simulink model "simulinkm2"  (R2020b)
settings: Solver=VariableStepAuto  StartTime=0.0  StopTime=10.0  RelTol=1e-3
(part 3 of 5)

== matlab function simulinkm2/MATLAB Function2 ==
  data: q input; V_F output; q_dot input
 function V_F = forward_velocity_kinematics(q, q_dot)
    
    q1 = q(1)
     q2 = q(2)
     q3 = q(3)
     q4 = q(4)
     q5 = q(5)
     q6 = q(6)
    JM = [ 10*sin((pi*q5)/180)*(cos((pi*q1)/180)*sin((pi*q4)/180) - cos((pi*q2)/180)*cos((pi*q3)/180)*cos((pi*q4)/180)*sin((pi*q1)/180) + cos((pi*q4)/180)*sin((pi*q1)/180)*sin((pi*q2)/180)*sin((pi*q3)/180)) - 5*cos((pi*q2)/180)*sin((pi*q1)/180) - 5*sin((pi*q1)/180) - 10*cos((pi*q2)/180)*sin((pi*q1)/180)*sin((pi*q3)/180) - 10*cos((pi*q3)/180)*sin((pi*q1)/180)*sin((pi*q2)/180) - 10*sin((pi*(q2 + q3))/180)*cos((pi*q5)/180)*sin((pi*q1)/180),                                                                                                                                                                                                                                                                                                                                                                                                                                                                                                                                                                                                                                                                  cos((pi*q1)/180)*(10*cos((pi*(q2 + q3))/180) - 5*sin((pi*q2)/180) - 5*sin((pi*(q2 + q3))/180)*sin((pi*(q4 + q5))/180) + 10*cos((pi*(q2 + q3))/180)*cos((pi*q5)/180) + 5*sin((pi*(q2 + q3))/180)*sin((pi*(q4 - q5))/180)),                                                                                                                                                                                                                                                                                                                                                                                                                                                                                                                                                                                                                                                                                                                                                                                                                         cos((pi*q1)/180)*(10*cos((pi*(q2 + q3))/180) - 5*sin((pi*(q2 + q3))/180)*sin((pi*(q4 + q5))/180) + 10*cos((pi*(q2 + q3))/180)*cos((pi*q5)/180) + 5*sin((pi*(q2 + q3))/180)*sin((pi*(q4 - q5))/180)),                                                                                                                                                                                                                                                                                                                           cos((pi*(q2 + q3))/180)*(5*sin((pi*q1)/180) + 5*cos((pi*q2)/180)*sin((pi*q1)/180) - 5*sin((pi*q1)/180)*(cos((pi*q2)/180) + 1) - 10*sin((pi*q5)/180)*(cos((pi*q1)/180)*sin((pi*q4)/180) - cos((pi*q2)/180)*cos((pi*q3)/180)*cos((pi*q4)/180)*sin((pi*q1)/180) + cos((pi*q4)/180)*sin((pi*q1)/180)*sin((pi*q2)/180)*sin((pi*q3)/180)) + 10*cos((pi*q2)/180)*sin((pi*q1)/180)*sin((pi*q3)/180) + 10*cos((pi*q3)/180)*sin((pi*q1)/180)*sin((pi*q2)/180) + 10*sin((pi*(q2 + q3))/180)*cos((pi*q5)/180)*sin((pi*q1)/180)) - sin((pi*(q2 + q3))/180)*sin((pi*q1)/180)*(10*cos((pi*(q2 + q3))/180) - 5*sin((pi*(q2 + q3))/180)*sin((pi*(q4 + q5))/180) + 10*cos((pi*(q2 + q3))/180)*cos((pi*q5)/180) + 5*sin((pi*(q2 + q3))/180)*sin((pi*(q4 - q5))/180)),                                                                                                                                                                                                                                                                                                                                                                                                                                                                                           (cos((pi*q1)/180)*cos((pi*q4)/180) - sin((pi*q4)/180)*(sin((pi*q1)/180)*sin((pi*q2)/180)*sin((pi*q3)/180) - cos((pi*q2)/180)*cos((pi*q3)/180)*sin((pi*q1)/180)))*(10*cos((pi*(q2 + q3))/180)*cos((pi*q5)/180) - 5*sin((pi*(q2 + q3))/180)*sin((pi*(q4 + q5))/180) + 5*sin((pi*(q2 + q3))/180)*sin((pi*(q4 - q5))/180)) + sin((pi*(q2 + q3))/180)*sin((pi*q4)/180)*(5*sin((pi*q1)/180) + 5*cos((pi*q2)/180)*sin((pi*q1)/180) - 5*sin((pi*q1)/180)*(2*sin((pi*(q2 + q3))/180) + cos((pi*q2)/180) + 1) - 10*sin((pi*q5)/180)*(cos((pi*q1)/180)*sin((pi*q4)/180) - cos((pi*q2)/180)*cos((pi*q3)/180)*cos((pi*q4)/180)*sin((pi*q1)/180) + cos((pi*q4)/180)*sin((pi*q1)/180)*sin((pi*q2)/180)*sin((pi*q3)/180)) + 10*cos((pi*q2)/180)*sin((pi*q1)/180)*sin((pi*q3)/180) + 10*cos((pi*q3)/180)*sin((pi*q1)/180)*sin((pi*q2)/180) + 10*sin((pi*(q2 + q3))/180)*cos((pi*q5)/180)*sin((pi*q1)/180)),                                                                                                                                                                                                                                                                                                                                                                                                                                                                                                                                                                             (cos((pi*(q2 + q3))/180)*cos((pi*q5)/180) - sin((pi*(q2 + q3))/180)*cos((pi*q4)/180)*sin((pi*q5)/180))*(5*sin((pi*q1)/180) + 5*cos((pi*q2)/180)*sin((pi*q1)/180) - 5*sin((pi*q1)/180)*(2*sin((pi*(q2 + q3))/180) + cos((pi*q2)/180) + 1) - 10*sin((pi*q5)/180)*(cos((pi*q1)/180)*sin((pi*q4)/180) - cos((pi*q2)/180)*cos((pi*q3)/180)*cos((pi*q4)/180)*sin((pi*q1)/180) + cos((pi*q4)/180)*sin((pi*q1)/180)*sin((pi*q2)/180)*sin((pi*q3)/180)) + 10*cos((pi*q2)/180)*sin((pi*q1)/180)*sin((pi*q3)/180) + 10*cos((pi*q3)/180)*sin((pi*q1)/180)*sin((pi*q2)/180) + 10*sin((pi*(q2 + q3))/180)*cos((pi*q5)/180)*sin((pi*q1)/180)) + (sin((pi*q5)/180)*(cos((pi*q4)/180)*(sin((pi*q1)/180)*sin((pi*q2)/180)*sin((pi*q3)/180) - cos((pi*q2)/180)*cos((pi*q3)/180)*sin((pi*q1)/180)) + cos((pi*q1)/180)*sin((pi*q4)/180)) - cos((pi*q5)/180)*(cos((pi*q2)/180)*sin((pi*q1)/180)*sin((pi*q3)/180) + cos((pi*q3)/180)*sin((pi*q1)/180)*sin((pi*q2)/180)))*(10*cos((pi*(q2 + q3))/180)*cos((pi*q5)/180) - 5*sin((pi*(q2 + q3))/180)*sin((pi*(q4 + q5))/180) + 5*sin((pi*(q2 + q3))/180)*sin((pi*(q4 - q5))/180));
 5*cos((pi*q1)/180) + 5*cos((pi*q1)/180)*cos((pi*q2)/180) + 10*sin((pi*q5)/180)*(sin((pi*q1)/180)*sin((pi*q4)/180) + cos((pi*q1)/180)*cos((pi*q2)/180)*cos((pi*q3)/180)*cos((pi*q4)/180) - cos((pi*q1)/180)*cos((pi*q4)/180)*sin((pi*q2)/180)*sin((pi*q3)/180)) + 10*sin((pi*(q2 + q3))/180)*cos((pi*q1)/180)*cos((pi*q5)/180) + 10*cos((pi*q1)/180)*cos((pi*q2)/180)*sin((pi*q3)/180) + 10*cos((pi*q1)/180)*cos((pi*q3)/180)*sin((pi*q2)/180),                                                                                                                                                                                                                                                                                                                                                                                                                                                                                                                                                                                                                                                                  sin((pi*q1)/180)*(10*cos((pi*(q2 + q3))/180) - 5*sin((pi*q2)/180) - 5*sin((pi*(q2 + q3))/180)*sin((pi*(q4 + q5))/180) + 10*cos((pi*(q2 + q3))/180)*cos((pi*q5)/180) + 5*sin((pi*(q2 + q3))/180)*sin((pi*(q4 - q5))/180)),                                                                                                                                                                                                                                                                                                                                                                                                                                                                                                                                                                                                                                                                                                                                                                                                                         sin((pi*q1)/180)*(10*cos((pi*(q2 + q3))/180) - 5*sin((pi*(q2 + q3))/180)*sin((pi*(q4 + q5))/180) + 10*cos((pi*(q2 + q3))/180)*cos((pi*q5)/180) + 5*sin((pi*(q2 + q3))/180)*sin((pi*(q4 - q5))/180)),                                                                                                                                                                                                                                                                                                                           sin((pi*(q2 + q3))/180)*cos((pi*q1)/180)*(10*cos((pi*(q2 + q3))/180) - 5*sin((pi*(q2 + q3))/180)*sin((pi*(q4 + q5))/180) + 10*cos((pi*(q2 + q3))/180)*cos((pi*q5)/180) + 5*sin((pi*(q2 + q3))/180)*sin((pi*(q4 - q5))/180)) - cos((pi*(q2 + q3))/180)*(5*cos((pi*q1)/180) + 5*cos((pi*q1)/180)*cos((pi*q2)/180) - 5*cos((pi*q1)/180)*(cos((pi*q2)/180) + 1) + 10*sin((pi*q5)/180)*(sin((pi*q1)/180)*sin((pi*q4)/180) + cos((pi*q1)/180)*cos((pi*q2)/180)*cos((pi*q3)/180)*cos((pi*q4)/180) - cos((pi*q1)/180)*cos((pi*q4)/180)*sin((pi*q2)/180)*sin((pi*q3)/180)) + 10*sin((pi*(q2 + q3))/180)*cos((pi*q1)/180)*cos((pi*q5)/180) + 10*cos((pi*q1)/180)*cos((pi*q2)/180)*sin((pi*q3)/180) + 10*cos((pi*q1)/180)*cos((pi*q3)/180)*sin((pi*q2)/180)),                                                                                                                                                                                                                                                                                                                                                                                                                                                                                           (sin((pi*q4)/180)*(cos((pi*q1)/180)*sin((pi*q2)/180)*sin((pi*q3)/180) - cos((pi*q1)/180)*cos((pi*q2)/180)*cos((pi*q3)/180)) + cos((pi*q4)/180)*sin((pi*q1)/180))*(10*cos((pi*(q2 + q3))/180)*cos((pi*q5)/180) - 5*sin((pi*(q2 + q3))/180)*sin((pi*(q4 + q5))/180) + 5*sin((pi*(q2 + q3))/180)*sin((pi*(q4 - q5))/180)) - sin((pi*(q2 + q3))/180)*sin((pi*q4)/180)*(5*cos((pi*q1)/180) + 5*cos((pi*q1)/180)*cos((pi*q2)/180) - 5*cos((pi*q1)/180)*(2*sin((pi*(q2 + q3))/180) + cos((pi*q2)/180) + 1) + 10*sin((pi*q5)/180)*(sin((pi*q1)/180)*sin((pi*q4)/180) + cos((pi*q1)/180)*cos((pi*q2)/180)*cos((pi*q3)/180)*cos((pi*q4)/180) - cos((pi*q1)/180)*cos((pi*q4)/180)*sin((pi*q2)/180)*sin((pi*q3)/180)) + 10*sin((pi*(q2 + q3))/180)*cos((pi*q1)/180)*cos((pi*q5)/180) + 10*cos((pi*q1)/180)*cos((pi*q2)/180)*sin((pi*q3)/180) + 10*cos((pi*q1)/180)*cos((pi*q3)/180)*sin((pi*q2)/180)),                                                                                                                                                                                                                                                                                                                                                                                                                                                                                                                                                                           - (sin((pi*q5)/180)*(cos((pi*q4)/180)*(cos((pi*q1)/180)*sin((pi*q2)/180)*sin((pi*q3)/180) - cos((pi*q1)/180)*cos((pi*q2)/180)*cos((pi*q3)/180)) - sin((pi*q1)/180)*sin((pi*q4)/180)) - cos((pi*q5)/180)*(cos((pi*q1)/180)*cos((pi*q2)/180)*sin((pi*q3)/180) + cos((pi*q1)/180)*cos((pi*q3)/180)*sin((pi*q2)/180)))*(10*cos((pi*(q2 + q3))/180)*cos((pi*q5)/180) - 5*sin((pi*(q2 + q3))/180)*sin((pi*(q4 + q5))/180) + 5*sin((pi*(q2 + q3))/180)*sin((pi*(q4 - q5))/180)) - (cos((pi*(q2 + q3))/180)*cos((pi*q5)/180) - sin((pi*(q2 + q3))/180)*cos((pi*q4)/180)*sin((pi*q5)/180))*(5*cos((pi*q1)/180) + 5*cos((pi*q1)/180)*cos((pi*q2)/180) - 5*cos((pi*q1)/180)*(2*sin((pi*(q2 + q3))/180) + cos((pi*q2)/180) + 1) + 10*sin((pi*q5)/180)*(sin((pi*q1)/180)*sin((pi*q4)/180) + cos((pi*q1)/180)*cos((pi*q2)/180)*cos((pi*q3)/180)*cos((pi*q4)/180) - cos((pi*q1)/180)*cos((pi*q4)/180)*sin((pi*q2)/180)*sin((pi*q3)/180)) + 10*sin((pi*(q2 + q3))/180)*cos((pi*q1)/180)*cos((pi*q5)/180) + 10*cos((pi*q1)/180)*cos((pi*q2)/180)*sin((pi*q3)/180) + 10*cos((pi*q1)/180)*cos((pi*q3)/180)*sin((pi*q2)/180));
                                                                                                                                                                                                                                                                                                                                                                                                                                             0, cos((pi*q1)/180)*(5*cos((pi*q1)/180)*cos((pi*q2)/180) + 10*sin((pi*q5)/180)*(sin((pi*q1)/180)*sin((pi*q4)/180) + cos((pi*q1)/180)*cos((pi*q2)/180)*cos((pi*q3)/180)*cos((pi*q4)/180) - cos((pi*q1)/180)*cos((pi*q4)/180)*sin((pi*q2)/180)*sin((pi*q3)/180)) + 10*sin((pi*(q2 + q3))/180)*cos((pi*q1)/180)*cos((pi*q5)/180) + 10*cos((pi*q1)/180)*cos((pi*q2)/180)*sin((pi*q3)/180) + 10*cos((pi*q1)/180)*cos((pi*q3)/180)*sin((pi*q2)/180)) + sin((pi*q1)/180)*(5*cos((pi*q2)/180)*sin((pi*q1)/180) - 10*sin((pi*q5)/180)*(cos((pi*q1)/180)*sin((pi*q4)/180) - cos((pi*q2)/180)*cos((pi*q3)/180)*cos((pi*q4)/180)*sin((pi*q1)/180) + cos((pi*q4)/180)*sin((pi*q1)/180)*sin((pi*q2)/180)*sin((pi*q3)/180)) + 10*cos((pi*q2)/180)*sin((pi*q1)/180)*sin((pi*q3)/180) + 10*cos((pi*q3)/180)*sin((pi*q1)/180)*sin((pi*q2)/180) + 10*sin((pi*(q2 + q3))/180)*cos((pi*q5)/180)*sin((pi*q1)/180)), sin((pi*q1)/180)*(5*sin((pi*q1)/180) + 5*cos((pi*q2)/180)*sin((pi*q1)/180) - 5*sin((pi*q1)/180)*(cos((pi*q2)/180) + 1) - 10*sin((pi*q5)/180)*(cos((pi*q1)/180)*sin((pi*q4)/180) - cos((pi*q2)/180)*cos((pi*q3)/180)*cos((pi*q4)/180)*sin((pi*q1)/180) + cos((pi*q4)/180)*sin((pi*q1)/180)*sin((pi*q2)/180)*sin((pi*q3)/180)) + 10*cos((pi*q2)/180)*sin((pi*q1)/180)*sin((pi*q3)/180) + 10*cos((pi*q3)/180)*sin((pi*q1)/180)*sin((pi*q2)/180) + 10*sin((pi*(q2 + q3))/180)*cos((pi*q5)/180)*sin((pi*q1)/180)) + cos((pi*q1)/180)*(5*cos((pi*q1)/180) + 5*cos((pi*q1)/180)*cos((pi*q2)/180) - 5*cos((pi*q1)/180)*(cos((pi*q2)/180) + 1) + 10*sin((pi*q5)/180)*(sin((pi*q1)/180)*sin((pi*q4)/180) + cos((pi*q1)/180)*cos((pi*q2)/180)*cos((pi*q3)/180)*cos((pi*q4)/180) - cos((pi*q1)/180)*cos((pi*q4)/180)*sin((pi*q2)/180)*sin((pi*q3)/180)) + 10*sin((pi*(q2 + q3))/180)*cos((pi*q1)/180)*cos((pi*q5)/180) + 10*cos((pi*q1)/180)*cos((pi*q2)/180)*sin((pi*q3)/180) + 10*cos((pi*q1)/180)*cos((pi*q3)/180)*sin((pi*q2)/180)), sin((pi*(q2 + q3))/180)*cos((pi*q1)/180)*(5*sin((pi*q1)/180) + 5*cos((pi*q2)/180)*sin((pi*q1)/180) - 5*sin((pi*q1)/180)*(cos((pi*q2)/180) + 1) - 10*sin((pi*q5)/180)*(cos((pi*q1)/180)*sin((pi*q4)/180) - cos((pi*q2)/180)*cos((pi*q3)/180)*cos((pi*q4)/180)*sin((pi*q1)/180) + cos((pi*q4)/180)*sin((pi*q1)/180)*sin((pi*q2)/180)*sin((pi*q3)/180)) + 10*cos((pi*q2)/180)*sin((pi*q1)/180)*sin((pi*q3)/180) + 10*cos((pi*q3)/180)*sin((pi*q1)/180)*sin((pi*q2)/180) + 10*sin((pi*(q2 + q3))/180)*cos((pi*q5)/180)*sin((pi*q1)/180)) - sin((pi*(q2 + q3))/180)*sin((pi*q1)/180)*(5*cos((pi*q1)/180) + 5*cos((pi*q1)/180)*cos((pi*q2)/180) - 5*cos((pi*q1)/180)*(cos((pi*q2)/180) + 1) + 10*sin((pi*q5)/180)*(sin((pi*q1)/180)*sin((pi*q4)/180) + cos((pi*q1)/180)*cos((pi*q2)/180)*cos((pi*q3)/180)*cos((pi*q4)/180) - cos((pi*q1)/180)*cos((pi*q4)/180)*sin((pi*q2)/180)*sin((pi*q3)/180)) + 10*sin((pi*(q2 + q3))/180)*cos((pi*q1)/180)*cos((pi*q5)/180) + 10*cos((pi*q1)/180)*cos((pi*q2)/180)*sin((pi*q3)/180) + 10*cos((pi*q1)/180)*cos((pi*q3)/180)*sin((pi*q2)/180)), (cos((pi*q1)/180)*cos((pi*q4)/180) - sin((pi*q4)/180)*(sin((pi*q1)/180)*sin((pi*q2)/180)*sin((pi*q3)/180) - cos((pi*q2)/180)*cos((pi*q3)/180)*sin((pi*q1)/180)))*(5*cos((pi*q1)/180) + 5*cos((pi*q1)/180)*cos((pi*q2)/180) - 5*cos((pi*q1)/180)*(2*sin((pi*(q2 + q3))/180) + cos((pi*q2)/180) + 1) + 10*sin((pi*q5)/180)*(sin((pi*q1)/180)*sin((pi*q4)/180) + cos((pi*q1)/180)*cos((pi*q2)/180)*cos((pi*q3)/180)*cos((pi*q4)/180) - cos((pi*q1)/180)*cos((pi*q4)/180)*sin((pi*q2)/180)*sin((pi*q3)/180)) + 10*sin((pi*(q2 + q3))/180)*cos((pi*q1)/180)*cos((pi*q5)/180) + 10*cos((pi*q1)/180)*cos((pi*q2)/180)*sin((pi*q3)/180) + 10*cos((pi*q1)/180)*cos((pi*q3)/180)*sin((pi*q2)/180)) + (sin((pi*q4)/180)*(cos((pi*q1)/180)*sin((pi*q2)/180)*sin((pi*q3)/180) - cos((pi*q1)/180)*cos((pi*q2)/180)*cos((pi*q3)/180)) + cos((pi*q4)/180)*sin((pi*q1)/180))*(5*sin((pi*q1)/180) + 5*cos((pi*q2)/180)*sin((pi*q1)/180) - 5*sin((pi*q1)/180)*(2*sin((pi*(q2 + q3))/180) + cos((pi*q2)/180) + 1) - 10*sin((pi*q5)/180)*(cos((pi*q1)/180)*sin((pi*q4)/180) - cos((pi*q2)/180)*cos((pi*q3)/180)*cos((pi*q4)/180)*sin((pi*q1)/180) + cos((pi*q4)/180)*sin((pi*q1)/180)*sin((pi*q2)/180)*sin((pi*q3)/180)) + 10*cos((pi*q2)/180)*sin((pi*q1)/180)*sin((pi*q3)/180) + 10*cos((pi*q3)/180)*sin((pi*q1)/180)*sin((pi*q2)/180) + 10*sin((pi*(q2 + q3))/180)*cos((pi*q5)/180)*sin((pi*q1)/180)), (sin((pi*q5)/180)*(cos((pi*q4)/180)*(sin((pi*q1)/180)*sin((pi*q2)/180)*sin((pi*q3)/180) - cos((pi*q2)/180)*cos((pi*q3)/180)*sin((pi*q1)/180)) + cos((pi*q1)/180)*sin((pi*q4)/180)) - cos((pi*q5)/180)*(cos((pi*q2)/180)*sin((pi*q1)/180)*sin((pi*q3)/180) + cos((pi*q3)/180)*sin((pi*q1)/180)*sin((pi*q2)/180)))*(5*cos((pi*q1)/180) + 5*cos((pi*q1)/180)*cos((pi*q2)/180) - 5*cos((pi*q1)/180)*(2*sin((pi*(q2 + q3))/180) + cos((pi*q2)/180) + 1) + 10*sin((pi*q5)/180)*(sin((pi*q1)/180)*sin((pi*q4)/180) + cos((pi*q1)/180)*cos((pi*q2)/180)*cos((pi*q3)/180)*cos((pi*q4)/180) - cos((pi*q1)/180)*cos((pi*q4)/180)*sin((pi*q2)/180)*sin((pi*q3)/180)) + 10*sin((pi*(q2 + q3))/180)*cos((pi*q1)/180)*cos((pi*q5)/180) + 10*cos((pi*q1)/180)*cos((pi*q2)/180)*sin((pi*q3)/180) + 10*cos((pi*q1)/180)*cos((pi*q3)/180)*sin((pi*q2)/180)) - (sin((pi*q5)/180)*(cos((pi*q4)/180)*(cos((pi*q1)/180)*sin((pi*q2)/180)*sin((pi*q3)/180) - cos((pi*q1)/180)*cos((pi*q2)/180)*cos((pi*q3)/180)) - sin((pi*q1)/180)*sin((pi*q4)/180)) - cos((pi*q5)/180)*(cos((pi*q1)/180)*cos((pi*q2)/180)*sin((pi*q3)/180) + cos((pi*q1)/180)*cos((pi*q3)/180)*sin((pi*q2)/180)))*(5*sin((pi*q1)/180) + 5*cos((pi*q2)/180)*sin((pi*q1)/180) - 5*sin((pi*q1)/180)*(2*sin((pi*(q2 + q3))/180) + cos((pi*q2)/180) + 1) - 10*sin((pi*q5)/180)*(cos((pi*q1)/180)*sin((pi*q4)/180) - cos((pi*q2)/180)*cos((pi*q3)/180)*cos((pi*q4)/180)*sin((pi*q1)/180) + cos((pi*q4)/180)*sin((pi*q1)/180)*sin((pi*q2)/180)*sin((pi*q3)/180)) + 10*cos((pi*q2)/180)*sin((pi*q1)/180)*sin((pi*q3)/180) + 10*cos((pi*q3)/180)*sin((pi*q1)/180)*sin((pi*q2)/180) + 10*sin((pi*(q2 + q3))/180)*cos((pi*q5)/180)*sin((pi*q1)/180));
                                                                                                                                                                                                                                                                                                                                                                                                                                             0,                                                                                                                                                                                                                                                                                                                                                                                                                                                                                                                                                                                                                                                                                                                                                                                                                                                                          sin((pi*q1)/180),                                                                                                                                                                                                                                                                                                                                                                                                                                                                                                                                                                                                                                                                                                                                                                                                                                                                                                                                                                                                            sin((pi*q1)/180),                                                                                                                                                                                                                                                                                                                                                                                                                                                                                                                                                                                                                                                                                                                                                                                                                                                                                                                                                                                                                                    sin((pi*(q2 + q3))/180)*cos((pi*q1)/180),                                                                                                                                                                                                                                                                                                                                                                                                                                                                                                                                                                                                                                                                                                                                                                                                                                                                                                                                                                                                                                                                                                                                                                                                                      sin((pi*q4)/180)*(cos((pi*q1)/180)*sin((pi*q2)/180)*sin((pi*q3)/180) - cos((pi*q1)/180)*cos((pi*q2)/180)*cos((pi*q3)/180)) + cos((pi*q4)/180)*sin((pi*q1)/180),                                                                                                                                                                                                                                                                                                                                                                                                                                                                                                                                                                                                                                                                                                                                                                                                                                                                                                                                                                                                                                                                                                                                                                                                                                                                                                                                                                      cos((pi*q5)/180)*(cos((pi*q1)/180)*cos((pi*q2)/180)*sin((pi*q3)/180) + cos((pi*q1)/180)*cos((pi*q3)/180)*sin((pi*q2)/180)) - sin((pi*q5)/180)*(cos((pi*q4)/180)*(cos((pi*q1)/180)*sin((pi*q2)/180)*sin((pi*q3)/180) - cos((pi*q1)/180)*cos((pi*q2)/180)*cos((pi*q3)/180)) - sin((pi*q1)/180)*sin((pi*q4)/180));
                                                                                                                                                                                                                                                                                                                                                                                                                                             0,                                                                                                                                                                                                                                                                                                                                                                                                                                                                                                                                                                                                                                                                                                                                                                                                                                                                         -cos((pi*q1)/180),                                                                                                                                                                                                                                                                                                                                                                                                                                                                                                                                                                                                                                                                                                                                                                                                                                                                                                                                                                                                           -cos((pi*q1)/180),                                                                                                                                                                                                                                                                                                                                                                                                                                                                                                                                                                                                                                                                                                                                                                                                                                                                                                                                                                                                                                    sin((pi*(q2 + q3))/180)*sin((pi*q1)/180),                                                                                                                                                                                                                                                                                                                                                                                                                                                                                                                                                                                                                                                                                                                                                                                                                                                                                                                                                                                                                                                                                                                                                                                                                      sin((pi*q4)/180)*(sin((pi*q1)/180)*sin((pi*q2)/180)*sin((pi*q3)/180) - cos((pi*q2)/180)*cos((pi*q3)/180)*sin((pi*q1)/180)) - cos((pi*q1)/180)*cos((pi*q4)/180),                                                                                                                                                                                                                                                                                                                                                                                                                                                                                                                                                                                                                                                                                                                                                                                                                                                                                                                                                                                                                                                                                                                                                                                                                                                                                                                                                                      cos((pi*q5)/180)*(cos((pi*q2)/180)*sin((pi*q1)/180)*sin((pi*q3)/180) + cos((pi*q3)/180)*sin((pi*q1)/180)*sin((pi*q2)/180)) - sin((pi*q5)/180)*(cos((pi*q4)/180)*(sin((pi*q1)/180)*sin((pi*q2)/180)*sin((pi*q3)/180) - cos((pi*q2)/180)*cos((pi*q3)/180)*sin((pi*q1)/180)) + cos((pi*q1)/180)*sin((pi*q4)/180));
                                                                                                                                                                                                                                                                                                                                                                                                                                             1,                                                                                                                                                                                                                                                                                                                                                                                                                                                                                                                                                                                                                                                                                                                                                                                                                                                                                         0,                                                                                                                                                                                                                                                                                                                                                                                                                                                                                                                                                                                                                                                                                                                                                                                                                                                                                                                                                                                                                           0,                                                                                                                                                                                                                                                                                                                                                                                                                                                                                                                                                                                                                                                                                                                                                                                                                                                                                                                                                                                                                                                    -cos((pi*(q2 + q3))/180),                                                                                                                                                                                                                                                                                                                                                                                                                                                                                                                                                                                                                                                                                                                                                                                                                                                                                                                                                                                                                                                                                                                                                                                                                                                                                                                                           -sin((pi*(q2 + q3))/180)*sin((pi*q4)/180),                                                                                                                                                                                                                                                                                                                                                                                                                                                                                                                                                                                                                                                                                                                                                                                                                                                                                                                                                                                                                                                                                                                                                                                                                                                                                                                                                                                                                                                                                                                                                                                sin((pi*(q2 + q3))/180)*cos((pi*q4)/180)*sin((pi*q5)/180) - cos((pi*(q2 + q3))/180)*cos((pi*q5)/180)]
                                                                                                                                                                                                                                                                                                                                                                                                                                         
                                                                                                                                                                                                                                                                                                                                                                                                                                         
                                                                                                                                                                                                                                                                                                                                                                                                                                         
  
   
   
   
   V_F= JM * q_dot
   
end
